simulink model "VFO_model"  (Simulink 8.7)
settings: Solver=VariableStepAuto  StartTime=0.0  StopTime=6  RelTol=1e-3
values from neighbouring files (symbols this model uses):
  J_1 = inv(J)    [Init.m]
  kc = 2*ki    (= 131.217957905)    [Init.m]
  ki = (T*omega_0^2)/(K*kp)    (= 65.6089789525)    [Init.m]
  Km = [km 0; 0 km]    [Init.m]
  kp = (2*T*zeta_0*omega_0 - 1)/K    (= 2.40689114415)    [Init.m]    (also in VFO_sciezka.m = 1)
  N_1 = inv(N)    [Init.m]
  Rm_1 = inv(Rm)    [Init.m]
  T_f = 1/ki    (= 0.0152418162265)    [Init.m]
  U_max = 9    [Init.m]
settings Model: Creator=Piotr  LastModifiedBy=Piotr
settings DataIOCC: LimitDataPoints=off  SaveFormat=Dataset
settings DebuggingCC: UnderspecifiedInitializationDetection=Simplified  MergeDetectMultiDrivingBlocksExec=error
settings HardwareCC: ProdBitPerPointer=64  ProdLargestAtomicFloat=Float  ProdIntDivRoundTo=Zero  ProdEndianess=LittleEndian  ProdWordSize=64  ProdHWDeviceType=Intel->x86-64 (Windows64)
settings ModelReferenceCC: PropagateSignalLabelsOutOfModel=on
settings ConfigComp: CovModelRefEnable=off

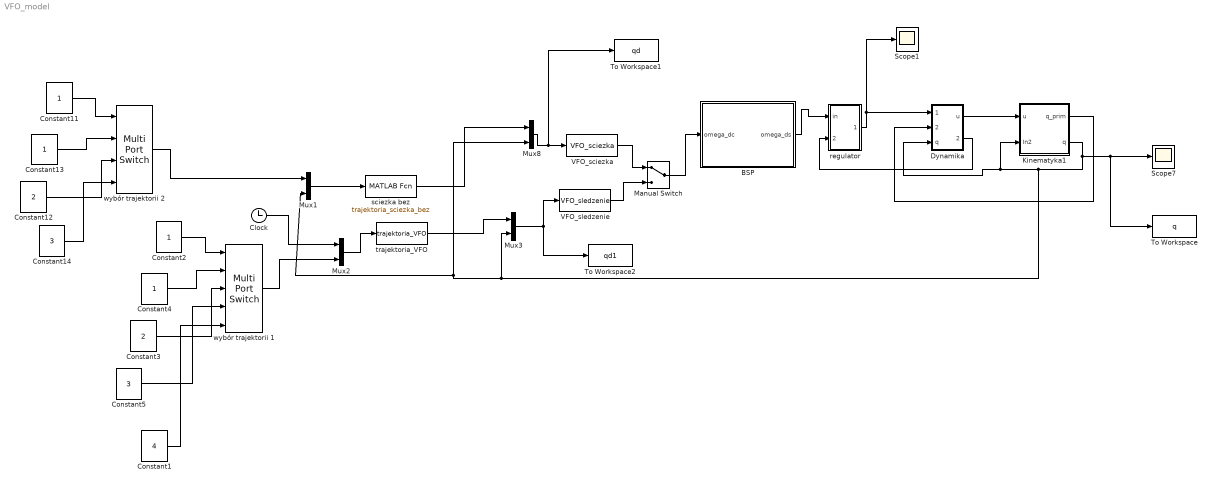
== system VFO_model ==
  BSP : Subsystem
  Clock : Clock
  Constant1 : Constant  Value=4
  Constant{2,4,11,13} (4 alike) : Constant
  Constant12 : Constant  Value=2
  Constant14 : Constant  Value=3
  Constant3 : Constant  Value=2
  Constant5 : Constant  Value=3
  Dynamika : Subsystem
  Kinematyka1 : Subsystem
  Manual Switch : ManualSwitch
  Mux{1..3,8} (4 alike) : Mux  Inputs=2
  Scope1 : Scope
  Scope7 : Scope
  To Workspace : ToWorkspace  VariableName=q  SampleTime=-1
  To Workspace1 : ToWorkspace  VariableName=qd  SampleTime=-1
  To Workspace2 : ToWorkspace  VariableName=qd1  SampleTime=-1
  VFO_sciezka : MATLABFcn  MATLABFcn=VFO_sciezka
  VFO_sledzenie : MATLABFcn  MATLABFcn=VFO_sledzenie
  regulator : Subsystem
  sciezka bez : MATLABFcn  MATLABFcn=trajektoria_sciezka_bez  OutputDimensions=6
  trajektoria_VFO : MATLABFcn  MATLABFcn=trajektoria_VFO  OutputDimensions=9
  wybór trajektorii 1 : MultiPortSwitch  Inputs=4
  wybór trajektorii 2 : MultiPortSwitch
  wires:
  Kinematyka1/2(q) -> To Workspace/1, Scope7/1, Mux3/2, Mux1/2, Mux8/2, Dynamika/3(q), Kinematyka1/2(In2)
  Kinematyka1/1(q_prim) -> Dynamika/2(qprim)
  Dynamika/1(u) -> Kinematyka1/1(u)
  regulator/1(Um) -> Scope1/1, Dynamika/1(Um)
  Dynamika/2(omega) -> regulator/2(In2)
  BSP/1(omega_ds) -> regulator/1(in)
  Constant11/1 -> wybór trajektorii 2/1
  Constant13/1 -> wybór trajektorii 2/2
  Constant12/1 -> wybór trajektorii 2/3
  Constant14/1 -> wybór trajektorii 2/4
  Mux1/1 -> sciezka bez/1
  Mux8/1 -> VFO_sciezka/1, To Workspace1/1
  sciezka bez/1 -> Mux8/1
  wybór trajektorii 2/1 -> Mux1/1
  Constant2/1 -> wybór trajektorii 1/1
  Constant4/1 -> wybór trajektorii 1/2
  Constant3/1 -> wybór trajektorii 1/3
  Constant5/1 -> wybór trajektorii 1/4
  Mux2/1 -> trajektoria_VFO/1
  Clock/1 -> Mux2/1
  wybór trajektorii 1/1 -> Mux2/2
  Mux3/1 -> VFO_sledzenie/1, To Workspace2/1
  trajektoria_VFO/1 -> Mux3/1
  VFO_sciezka/1 -> Manual Switch/1
  VFO_sledzenie/1 -> Manual Switch/2
  Manual Switch/1 -> BSP/1(omega_dc)
  Constant1/1 -> wybór trajektorii 1/5

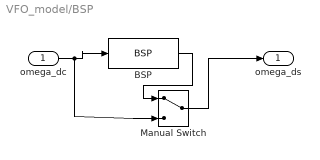
== system VFO_model/BSP ==
  omega_dc : Inport
  BSP : MATLABFcn  MATLABFcn=BSP
  Manual Switch : ManualSwitch
  omega_ds : Outport
  wires:
  BSP/1 -> Manual Switch/1
  omega_dc/1 -> Manual Switch/2, BSP/1
  Manual Switch/1 -> omega_ds/1

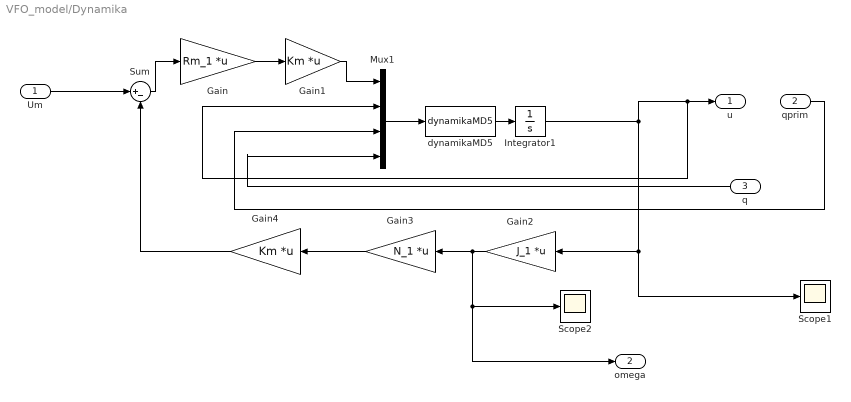
== system VFO_model/Dynamika ==
  Um : Inport
  qprim : Inport  Port=2
  q : Inport  Port=3
  Gain : Gain  Gain=Rm_1  Multiplication=Matrix(K*u)
  Gain1 : Gain  Gain=Km  Multiplication=Matrix(K*u)
  Gain2 : Gain  Gain=J_1  Multiplication=Matrix(K*u)
  Gain3 : Gain  Gain=N_1  Multiplication=Matrix(K*u)
  Gain4 : Gain  Gain=Km  Multiplication=Matrix(K*u)
  Integrator1 : Integrator  InitialCondition=[0 0]
  Mux1 : Mux
  Scope1 : Scope
  Scope2 : Scope
  Sum : Sum  Inputs=|+-
  "dynamikaMD5 " : MATLABFcn  MATLABFcn=dynamikaMD5
  u : Outport
  omega : Outport  Port=2
  wires:
  "dynamikaMD5 "/1 -> Integrator1/1
  Gain/1 -> Gain1/1
  Gain3/1 -> Gain4/1
  Mux1/1 -> "dynamikaMD5 "/1
  Um/1 -> Sum/1
  Gain4/1 -> Sum/2
  Gain1/1 -> Mux1/1
  Sum/1 -> Gain/1
  Integrator1/1 -> u/1, Mux1/2, Scope1/1, Gain2/1
  qprim/1 -> Mux1/3
  Gain2/1 -> Scope2/1, omega/1, Gain3/1
  q/1 -> Mux1/4

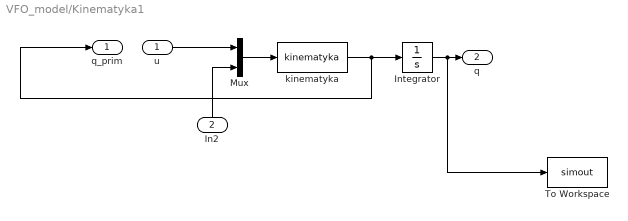
== system VFO_model/Kinematyka1 ==
  u : Inport
  In2 : Inport  Port=2
  Integrator : Integrator  InitialCondition=[0;0.1;0]
  Mux : Mux  Inputs=2
  To Workspace : ToWorkspace  VariableName=simout  SampleTime=-1
  kinematyka : MATLABFcn  MATLABFcn=kinematyka
  q_prim : Outport
  q : Outport  Port=2
  wires:
  In2/1 -> Mux/2
  kinematyka/1 -> q_prim/1, Integrator/1
  Integrator/1 -> To Workspace/1, q/1
  Mux/1 -> kinematyka/1
  u/1 -> Mux/1

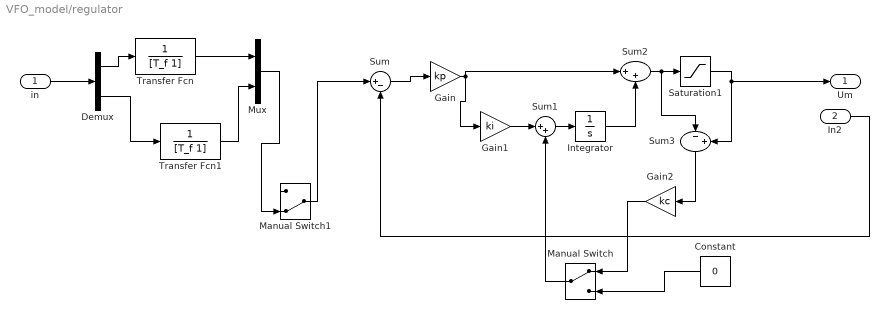
== system VFO_model/regulator ==
  in : Inport
  In2 : Inport  Port=2
  Constant : Constant  Value=0
  Demux : Demux  Outputs=2
  Gain : Gain  Gain=kp
  Gain1 : Gain  Gain=ki
  Gain2 : Gain  Gain=kc
  Integrator : Integrator
  Manual Switch : ManualSwitch
  Manual Switch1 : ManualSwitch  CurrentSetting=0
  Mux : Mux  Inputs=2
  Saturation1 : Saturate  UpperLimit=U_max  LowerLimit=-U_max
  Sum : Sum  Inputs=|+-
  Sum1 : Sum  Inputs=|++
  Sum2 : Sum  Inputs=|++
  Sum3 : Sum  Inputs=|-+
  Transfer Fcn : TransferFcn  Denominator=[T_f 1]
  Transfer Fcn1 : TransferFcn  Denominator=[T_f 1]
  Um : Outport
  wires:
  Integrator/1 -> Sum2/2
  Sum2/1 -> Sum3/1, Saturation1/1
  Sum1/1 -> Integrator/1
  Saturation1/1 -> Um/1, Sum3/2
  Sum3/1 -> Gain2/1
  Gain1/1 -> Sum1/1
  In2/1 -> Sum/2
  Sum/1 -> Gain/1
  Gain/1 -> Sum2/1, Gain1/1
  in/1 -> Demux/1
  Mux/1 -> Manual Switch1/2
  Gain2/1 -> Manual Switch/1
  Constant/1 -> Manual Switch/2
  Manual Switch/1 -> Sum1/2
  Demux/1 -> Transfer Fcn/1
  Transfer Fcn/1 -> Mux/1
  Demux/2 -> Transfer Fcn1/1
  Transfer Fcn1/1 -> Mux/2
  Manual Switch1/1 -> Sum/1
